simulink model "Q2_M1"  (R2024b)
settings: Solver=VariableStepAuto  StartTime=0.0  StopTime=10.0  RelTol=1e-3
settings Model: Creator=chall  LastModifiedBy=chall

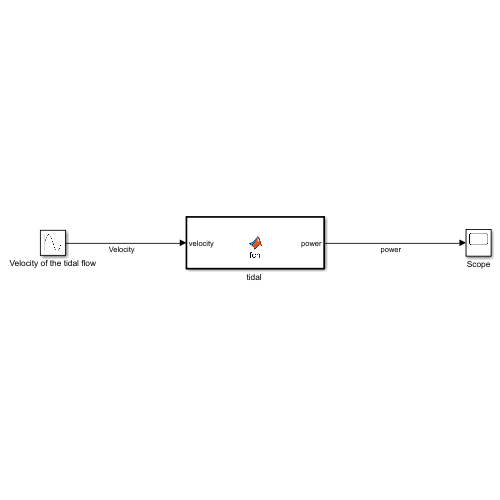
[thumbnail: Simulink's stored preview of the top-level diagram]
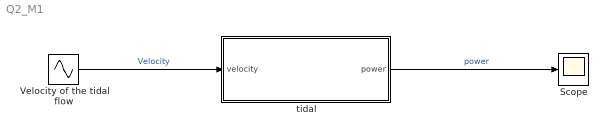
== system Q2_M1 ==
  Scope : Scope
  Velocity of the tidal flow : Sin  SampleTime=0
  "tidal " : MATLAB Function  TreatAsAtomicUnit=on
  wires:
  Velocity of the tidal flow/1 -> "tidal "/1(velocity)  "Velocity"
  "tidal "/1(power) -> Scope/1  "power"

== matlab function Q2_M1/tidal  ==
  data: velocity input; power output
function power = fcn(velocity)

 power = 0.5*1025*100*velocity^3;
end
